simulink model "satellite_attitude_sun_mode_model"  (R2017a)
settings: Solver=ode4  StartTime=0.0  StopTime=tdur  FixedStep=dt  RelTol=1e-3  EnableMultiTasking=on
undefined symbols (not defined in the file or in its folder): alpha_dem, beta_dem, Kdx, Kdy, Kdz, Kpx, Kpy, Krcs, q_bi0, rate_dem_x, rate_dem_y, rate_dem_z, rate_sensor_model_type, s_i, sigma_w, sun_sensor_model_type, T_env, ta, Tdb, tdelay, Trcs_saturation, w_bi0, w_bias
settings Model: Creator=Goh  LastModifiedBy=Rusty Goh
settings DataIOCC: SaveFormat=Array
settings OptimizationCC: LifeSpan=inf
settings DebuggingCC: UnderspecifiedInitializationDetection=Classic  MergeDetectMultiDrivingBlocksExec=none  StateNameClashWarn=warning  SFUnexpectedBacktrackingDiag=warning  SFNoUnconditionalDefaultTransitionDiag=warning  SFExecutionAtInitializationDiag=none
settings HardwareCC: ProdBitPerPointer=32  ProdBitPerSizeT=32  ProdBitPerPtrDiffT=32  ProdLargestAtomicFloat=None  ProdIntDivRoundTo=Undefined  ProdEndianess=Unspecified  ProdWordSize=32  ProdHWDeviceType=32-bit Generic
settings ModelReferenceCC: PropagateSignalLabelsOutOfModel=off
settings GRTTargetCC: TargetLangStandard=C89/C90 (ANSI)  GeneratePreprocessorConditionals=Disable all
settings ConfigComp: CovMetricSettings=dw  CovHtmlReporting=on  CovSaveCumulativeToWorkspaceVar=on  CovSaveSingleToWorkspaceVar=on  CovExternalEMLEnable=off

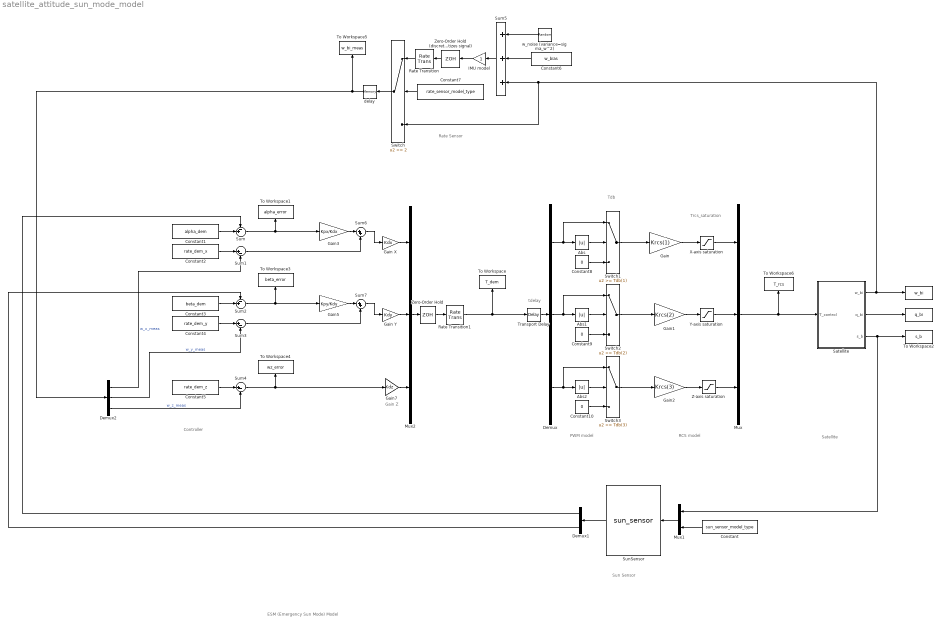
== system satellite_attitude_sun_mode_model ==
  note: Gain Z
  note: tdelay
  note: Trcs_saturation
  note: Tdb
  note: Satellite
  note: Sun Sensor
  note: Rate Sensor
  note: Controller
  note: PWM model
  note: RCS model
  note: ESM (Emergency Sun Mode) Model
  " " : ToWorkspace  VariableName=w_bi  SampleTime=-1
  "  " : ToWorkspace  VariableName=q_bi  SampleTime=-1
  Abs : Abs  SaturateOnIntegerOverflow=on
  Abs1 : Abs  SaturateOnIntegerOverflow=on
  Abs2 : Abs  SaturateOnIntegerOverflow=on
  Constant : Constant  Value=sun_sensor_model_type
  Constant1 : Constant  Value=alpha_dem
  Constant10 : Constant  Value=0
  Constant2 : Constant  Value=rate_dem_x
  Constant3 : Constant  Value=beta_dem
  Constant4 : Constant  Value=rate_dem_y
  Constant5 : Constant  Value=rate_dem_z
  Constant6 : Constant  Value=w_bias
  Constant7 : Constant  Value=rate_sensor_model_type
  Constant8 : Constant  Value=0
  Constant9 : Constant  Value=0
  Demux : Demux  Outputs=3
  Demux1 : Demux  Outputs=2
  Demux2 : Demux  Outputs=3
  Gain : Gain  Gain=Krcs(1)  SaturateOnIntegerOverflow=on  OutDataTypeStr=Inherit: Same as input  ParamDataTypeStr=Inherit: Same as input
  Gain X : Gain  Gain=Kdx
  Gain Y : Gain  Gain=Kdy
  Gain1 : Gain  Gain=Krcs(2)  SaturateOnIntegerOverflow=on  OutDataTypeStr=Inherit: Same as input  ParamDataTypeStr=Inherit: Same as input
  Gain2 : Gain  Gain=Krcs(3)  SaturateOnIntegerOverflow=on  OutDataTypeStr=Inherit: Same as input  ParamDataTypeStr=Inherit: Same as input
  Gain3 : Gain  Gain=Kpx/Kdx
  Gain5 : Gain  Gain=Kpy/Kdy
  Gain7 : Gain  Gain=Kdz  SaturateOnIntegerOverflow=on  OutDataTypeStr=Inherit: Same as input  ParamDataTypeStr=Inherit: Same as input
  IMU model : Gain  SaturateOnIntegerOverflow=on  OutDataTypeStr=Inherit: Same as input  ParamDataTypeStr=Inherit: Same as input
  Mux : Mux  Inputs=3
  Mux1 : Mux  Inputs=2
  Mux2 : Mux  Inputs=3
  Rate Transition : RateTransition
  Rate Transition1 : RateTransition
  Satellite : Subsystem
  Sum : Sum  Inputs=-+|  SaturateOnIntegerOverflow=on
  Sum1 : Sum  Inputs=|+-  SaturateOnIntegerOverflow=on
  Sum2 : Sum  Inputs=-+|  SaturateOnIntegerOverflow=on
  Sum3 : Sum  Inputs=|+-  SaturateOnIntegerOverflow=on
  Sum4 : Sum  Inputs=|+-  SaturateOnIntegerOverflow=on
  Sum5 : Sum  Inputs=+++  SaturateOnIntegerOverflow=on
  Sum6 : Sum  Inputs=|++
  Sum7 : Sum  Inputs=|++
  SunSensor : MATLABFcn  MATLABFcn=sun_sensor  OutputDimensions=2
  Switch : Switch  Threshold=2  SaturateOnIntegerOverflow=on
  Switch1 : Switch  Threshold=Tdb(1)  SaturateOnIntegerOverflow=on
  Switch2 : Switch  Threshold=Tdb(2)  SaturateOnIntegerOverflow=on
  Switch3 : Switch  Threshold=Tdb(3)  SaturateOnIntegerOverflow=on
  To Workspace : ToWorkspace  VariableName=T_dem  SampleTime=-1
  To Workspace1 : ToWorkspace  VariableName=alpha_error  SampleTime=-1
  To Workspace2 : ToWorkspace  VariableName=s_b  SampleTime=-1
  To Workspace3 : ToWorkspace  VariableName=beta_error  SampleTime=-1
  To Workspace4 : ToWorkspace  VariableName=wz_error  SampleTime=-1
  To Workspace5 : ToWorkspace  VariableName=w_bi_meas  SampleTime=-1
  To Workspace6 : ToWorkspace  VariableName=T_rcs  SampleTime=-1
  Transport Delay : TransportDelay  DelayTime=tdelay
  X-axis saturation : Saturate  UpperLimit=+Trcs_saturation(1)  LowerLimit=-Trcs_saturation(1)
  Y-axis saturation : Saturate  UpperLimit=+Trcs_saturation(2)  LowerLimit=-Trcs_saturation(2)
  Z-axis saturation : Saturate  UpperLimit=+Trcs_saturation(3)  LowerLimit=-Trcs_saturation(3)
  Zero-Order Hold : ZeroOrderHold  SampleTime=ta
  Zero-Order Hold (discretetizes signal) : ZeroOrderHold  SampleTime=ta
  delay : Memory
  w_noise (variance=sigma_w^2) : RandomNumber  Variance=sigma_w^2  SampleTime=0
  wires:
  Mux/1 -> To Workspace6/1, Satellite/1(T_control)
  Satellite/2(q_bi) -> "  "/1
  X-axis saturation/1 -> Mux/1
  Y-axis saturation/1 -> Mux/2
  Z-axis saturation/1 -> Mux/3
  Transport Delay/1 -> Demux/1
  Switch1/1 -> Gain/1
  Gain/1 -> X-axis saturation/1
  Gain1/1 -> Y-axis saturation/1
  Gain2/1 -> Z-axis saturation/1
  Satellite/3(s_b) -> Mux1/1, To Workspace2/1
  Mux1/1 -> SunSensor/1
  Constant/1 -> Mux1/2
  SunSensor/1 -> Demux1/1
  Sum/1 -> Gain3/1, To Workspace1/1
  Constant2/1 -> Sum1/1
  Sum1/1 -> Sum6/2
  Constant1/1 -> Sum/2
  Sum2/1 -> Gain5/1, To Workspace3/1
  Constant4/1 -> Sum3/1
  Constant3/1 -> Sum2/2
  Demux1/1 -> Sum/1
  Gain X/1 -> Mux2/1
  Demux2/1 -> Sum1/2  "w_x_meas"
  Demux2/2 -> Sum3/2  "w_y_meas"
  Mux2/1 -> Zero-Order Hold/1
  delay/1 -> Demux2/1, To Workspace5/1
  Demux1/2 -> Sum2/1
  Demux2/3 -> Sum4/2  "w_z_meas"
  Sum4/1 -> Gain7/1, To Workspace4/1
  Constant5/1 -> Sum4/1
  Gain7/1 -> Mux2/3
  IMU model/1 -> Zero-Order Hold (discretetizes signal)/1
  w_noise (variance=sigma_w^2)/1 -> Sum5/1
  Sum5/1 -> IMU model/1
  Constant6/1 -> Sum5/2
  Satellite/1(w_bi) -> " "/1, Switch/3, Sum5/3
  Switch/1 -> delay/1
  Constant7/1 -> Switch/2
  Gain3/1 -> Sum6/1
  Sum6/1 -> Gain X/1
  Sum3/1 -> Sum7/2
  Gain5/1 -> Sum7/1
  Sum7/1 -> Gain Y/1
  Gain Y/1 -> Mux2/2
  Abs/1 -> Switch1/2
  Constant8/1 -> Switch1/3
  Demux/1 -> Abs/1, Switch1/1
  Abs1/1 -> Switch2/2
  Constant9/1 -> Switch2/3
  Switch2/1 -> Gain1/1
  Abs2/1 -> Switch3/2
  Constant10/1 -> Switch3/3
  Demux/3 -> Switch3/1, Abs2/1
  Switch3/1 -> Gain2/1
  Demux/2 -> Switch2/1, Abs1/1
  Zero-Order Hold (discretetizes signal)/1 -> Rate Transition/1
  Rate Transition/1 -> Switch/1
  Zero-Order Hold/1 -> Rate Transition1/1
  Rate Transition1/1 -> To Workspace/1, Transport Delay/1

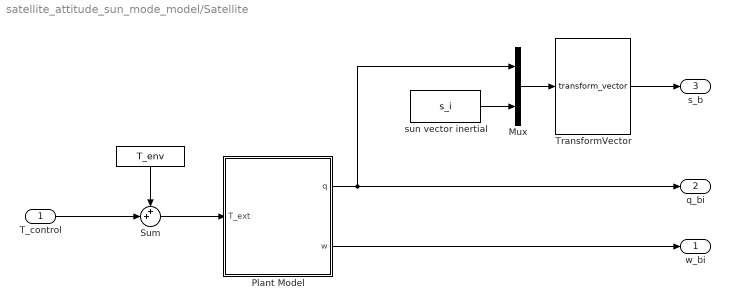
== system satellite_attitude_sun_mode_model/Satellite ==
  T_control : Inport
  " " : Constant  Value=T_env
  Mux : Mux  Inputs=2
  Plant Model : Subsystem
  Sum : Sum  Inputs=++|
  TransformVector : MATLABFcn  MATLABFcn=transform_vector
  sun vector inertial : Constant  Value=s_i
  w_bi : Outport
  q_bi : Outport  Port=2
  s_b : Outport  Port=3
  wires:
  Sum/1 -> Plant Model/1(T_ext)
  T_control/1 -> Sum/2
  Plant Model/2(w) -> w_bi/1
  Plant Model/1(q) -> Mux/1, q_bi/1
  " "/1 -> Sum/1
  TransformVector/1 -> s_b/1
  Mux/1 -> TransformVector/1
  sun vector inertial/1 -> Mux/2

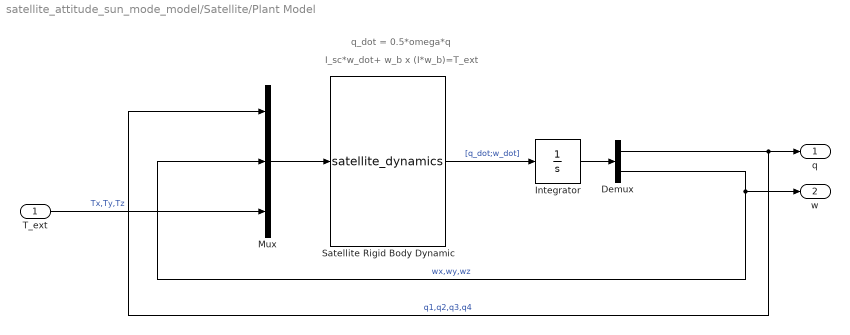
== system satellite_attitude_sun_mode_model/Satellite/Plant Model ==
  note: q_dot = 0.5*omega*q
  note: I_sc*w_dot+ w_b x (I*w_b)=T_ext
  T_ext : Inport
  Demux : Demux  Outputs=[4 3]
  Integrator : Integrator  InitialCondition=[q_bi0;w_bi0]
  Mux : Mux  Inputs=[4 3 3]
  Satellite Rigid Body Dynamic : MATLABFcn  MATLABFcn=satellite_dynamics  OutputDimensions=7
  q : Outport
  w : Outport  Port=2
  wires:
  Integrator/1 -> Demux/1
  T_ext/1 -> Mux/3  "Tx,Ty,Tz"
  Mux/1 -> Satellite Rigid Body Dynamic/1
  Demux/2 -> Mux/2, w/1  "wx,wy,wz"
  Demux/1 -> q/1, Mux/1  "q1,q2,q3,q4"
  Satellite Rigid Body Dynamic/1 -> Integrator/1  "[q_dot;w_dot]"
